simulink library "navigations"  (R2014a)
settings: Solver=ode45  StartTime=0.0  StopTime=10.0  RelTol=1e-3
undefined symbols (not defined in the file or in its folder): fdesignblkfcn, gcbh
libraries: simulink x8, visionstatistics x6
settings Model: Creator=jsustare  LastModifiedBy=jsustare

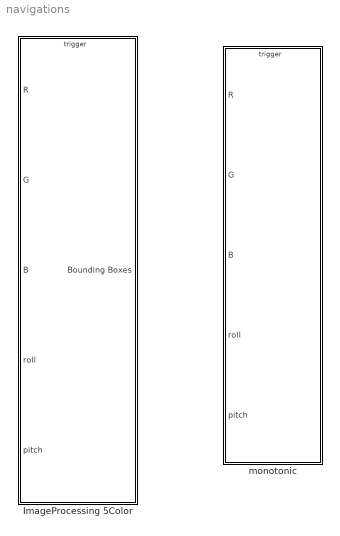
== system navigations ==
  ImageProcessing 5Color : Subsystem  TreatAsAtomicUnit=on  mask{blueThreshold=15, redThreshold=50, greenThreshold=50, yellowThreshold=160, purpleThreshold=160}
  monotonic : Subsystem  mask{whiteThreshold=0}
      mask prompts: whiteThreshold "whyite"

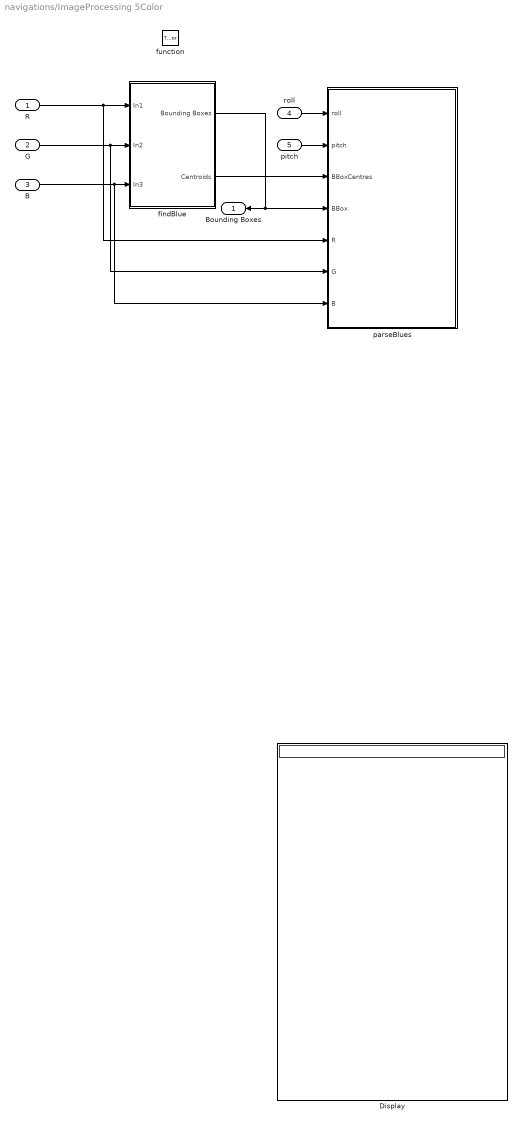
== system navigations/ImageProcessing 5Color ==
  R : Inport
  G : Inport  Port=2
  B : Inport  Port=3
  roll : Inport  Port=4
  pitch : Inport  Port=5
  function : TriggerPort  TriggerType=function-call
  Display : Display
  findBlue : Subsystem
  parseBlues : Subsystem  TreatAsAtomicUnit=on
  "Bounding Boxes " : Outport
  wires:
  pitch/1 -> parseBlues/2(pitch)
  roll/1 -> parseBlues/1(roll)
  findBlue/2(Centroids) -> parseBlues/3(BBoxCentres)
  findBlue/1(Bounding Boxes) -> "Bounding Boxes "/1, parseBlues/4(BBox)
  B/1 -> findBlue/3(In3), parseBlues/7(B)
  R/1 -> findBlue/1(In1), parseBlues/5(R)
  G/1 -> findBlue/2(In2), parseBlues/6(G)

== system navigations/monotonic ==
  note: use the writePos to store final positions per
      | landmark. keep inmind that this is suppose to
      |  beinside a loop and then the -1 scenarious would
      |  leand to -1000 cases
  R : Inport
  G : Inport  Port=2
  B : Inport  Port=3
  roll : Inport  Port=4
  pitch : Inport  Port=5
  function : TriggerPort  TriggerType=function-call
  MATLAB Function2 : MATLAB Function  TreatAsAtomicUnit=on
  detectLandMarks : Subsystem
  getPosition : Subsystem
  wires:
  R/1 -> detectLandMarks/1(R)
  B/1 -> detectLandMarks/3(B)
  G/1 -> detectLandMarks/2(G)

== system navigations/ImageProcessing 5Color/findBlue ==
  In1 : Inport
  In2 : Inport  Port=2
  In3 : Inport  Port=3
  Blob Analysis : visionstatistics/Blob Analysis  Tag=vipblks_row_conv  area=on  centroid=on  bBox=on  majorAxis=off  minorAxis=off  angle=off  eccentricity=off  equivDiameterSq=off  extent=off  perimeter=off  maxBlobs=16  warnIfNumBlobsExceeded=on  isCount=off  useMinArea=on  minArea=300  useMaxArea=off  maxArea=intmax('uint32')  excludeBorderBlob=on  outDT=double  isOutVarDim=off  isFill=on  fillValues=-1  conn=8  isLabel=off  outputMode=Binary point scaling  outputWordLength=32  outputFracLength=16  firstCoeffMode=Binary point scaling  firstCoeffWordLength=16  firstCoeffFracLength=14  secondCoeffMode=Binary point scaling  secondCoeffWordLength=32  secondCoeffFracLength=16  accumMode=Binary point scaling  accumWordLength=32  accumFracLength=0  prodOutputMode=Binary point scaling  prodOutputWordLength=32  prodOutputFracLength=16  roundingMode=Floor  overflowMode=off
  Compare To Constant : simulink/Logic and Bit Operations/Compare To Constant  relop=>  const=blueThreshold  OutDataTypeStr=boolean
  MATLAB Function : MATLAB Function  TreatAsAtomicUnit=on
  MATLAB Function1 : MATLAB Function  TreatAsAtomicUnit=on
  Bounding Boxes : Outport
  Centroids : Outport  Port=2
  wires:
  In3/1 -> MATLAB Function1/3(B)
  In2/1 -> MATLAB Function1/2(G)
  In1/1 -> MATLAB Function1/1(R)
  MATLAB Function1/1(blueIntensity) -> Compare To Constant/1
  Blob Analysis/2 -> MATLAB Function/2(centroid)
  MATLAB Function/1(centroid_largest) -> Centroids/1
  MATLAB Function/2(bbox_largest) -> Bounding Boxes/1
  Blob Analysis/1 -> MATLAB Function/1(area)
  Blob Analysis/3 -> MATLAB Function/3(bbox)
  Compare To Constant/1 -> Blob Analysis/1

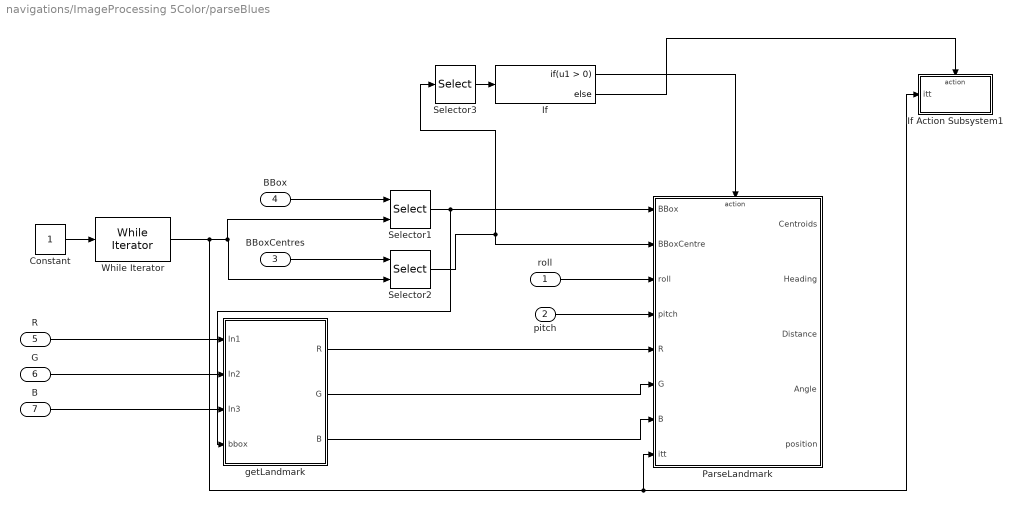
== system navigations/ImageProcessing 5Color/parseBlues ==
  roll : Inport
  pitch : Inport  Port=2
  BBoxCentres : Inport  Port=3
  BBox : Inport  Port=4
  R : Inport  Port=5
  G : Inport  Port=6
  B : Inport  Port=7
  Constant : Constant
  If : If
  If Action Subsystem1 : Subsystem  TreatAsAtomicUnit=on
  ParseLandmark : Subsystem  TreatAsAtomicUnit=on
  Selector1 : Selector  NumberOfDimensions=2  InputPortWidth=3  IndexOptions=Index vector (port),Select all  Indices=[1 3],1  OutputSizes=1,1
  Selector2 : Selector  NumberOfDimensions=2  InputPortWidth=3  IndexOptions=Index vector (port),Select all  Indices=[1 3],1  OutputSizes=1,1
  Selector3 : Selector  InputPortWidth=2
  While Iterator : WhileIterator  MaxIters=4  WhileBlockType=do-while  ShowIterationPort=on
  getLandmark : Subsystem
  wires:
  Selector3/1 -> If/1
  If/2 -> If Action Subsystem1/Action
  If/1 -> ParseLandmark/Action
  getLandmark/3(B) -> ParseLandmark/7(B)
  getLandmark/2(G) -> ParseLandmark/6(G)
  getLandmark/1(R) -> ParseLandmark/5(R)
  Constant/1 -> While Iterator/1
  B/1 -> getLandmark/3(In3)
  G/1 -> getLandmark/2(In2)
  R/1 -> getLandmark/1(In1)
  Selector2/1 -> ParseLandmark/2(BBoxCentre), Selector3/1
  Selector1/1 -> getLandmark/4(bbox), ParseLandmark/1(BBox)
  BBoxCentres/1 -> Selector2/1
  BBox/1 -> Selector1/1
  While Iterator/1 -> Selector2/2, Selector1/2, If Action Subsystem1/1(itt), ParseLandmark/8("itt ")
  pitch/1 -> ParseLandmark/4(pitch)
  roll/1 -> ParseLandmark/3(roll)

== system navigations/monotonic/detectLandMarks ==
  R : Inport
  G : Inport  Port=2
  B : Inport  Port=3
  Blob Analysis : visionstatistics/Blob Analysis  Tag=vipblks_row_conv  area=on  centroid=on  bBox=off  majorAxis=off  minorAxis=off  angle=off  eccentricity=off  equivDiameterSq=off  extent=off  perimeter=off  maxBlobs=16  warnIfNumBlobsExceeded=on  isCount=off  useMinArea=on  minArea=300  useMaxArea=off  maxArea=intmax('uint32')  excludeBorderBlob=on  outDT=double  isOutVarDim=off  isFill=on  fillValues=-1  conn=8  isLabel=off  outputMode=Binary point scaling  outputWordLength=32  outputFracLength=16  firstCoeffMode=Binary point scaling  firstCoeffWordLength=16  firstCoeffFracLength=14  secondCoeffMode=Binary point scaling  secondCoeffWordLength=32  secondCoeffFracLength=16  accumMode=Binary point scaling  accumWordLength=32  accumFracLength=0  prodOutputMode=Binary point scaling  prodOutputWordLength=32  prodOutputFracLength=16  roundingMode=Floor  overflowMode=off
  Compare To Constant : simulink/Logic and Bit Operations/Compare To Constant  relop=>  const=whiteThreshold  OutDataTypeStr=boolean
  MATLAB Function1 : MATLAB Function  TreatAsAtomicUnit=on
  MATLAB Function2 : MATLAB Function  TreatAsAtomicUnit=on
  centroids : Outport
  areas : Outport  Port=2
  wires:
  MATLAB Function1/2(areas_largest) -> areas/1
  MATLAB Function1/1(centroid_largest) -> centroids/1
  MATLAB Function2/1(whiteIntensity) -> Compare To Constant/1
  Blob Analysis/2 -> MATLAB Function1/2(centroid)
  Blob Analysis/1 -> MATLAB Function1/1(area)
  Compare To Constant/1 -> Blob Analysis/1
  B/1 -> MATLAB Function2/3(B)
  G/1 -> MATLAB Function2/2(G)
  R/1 -> MATLAB Function2/1(R)

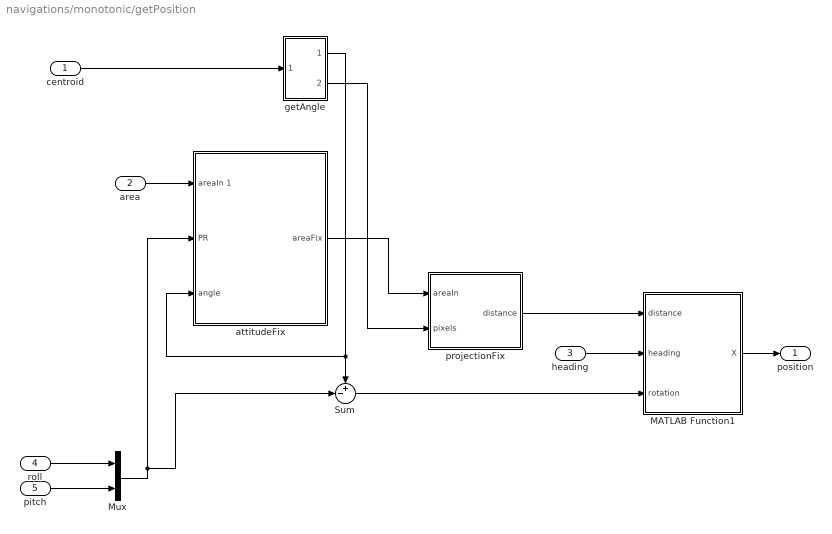
== system navigations/monotonic/getPosition ==
  centroid : Inport
  area : Inport  Port=2
  heading : Inport  Port=3
  "roll " : Inport  Port=4
  pitch : Inport  Port=5
  MATLAB Function1 : MATLAB Function  TreatAsAtomicUnit=on
  Mux : Mux  Inputs=2
  Sum : Sum  Inputs=+-|
  attitudeFix : Subsystem
  getAngle : Subsystem
  projectionFix : Subsystem
  position : Outport
  wires:
  getAngle/2(pixels) -> projectionFix/2(pixels)
  area/1 -> attitudeFix/1(areaIn 1)
  MATLAB Function1/1(X) -> position/1
  heading/1 -> MATLAB Function1/2(heading)
  projectionFix/1(distance) -> MATLAB Function1/1(distance)
  attitudeFix/1(areaFix) -> projectionFix/1(areaIn)
  Sum/1 -> MATLAB Function1/3(rotation)
  getAngle/1(angleRad) -> Sum/1, attitudeFix/3("angle ")
  Mux/1 -> Sum/2, attitudeFix/2(PR)
  pitch/1 -> Mux/2
  "roll "/1 -> Mux/1
  centroid/1 -> getAngle/1(centroid)

== system navigations/ImageProcessing 5Color/parseBlues/If Action Subsystem1 ==
  itt : Inport
  Action Port : ActionPort
  MATLAB Function1 : MATLAB Function  TreatAsAtomicUnit=on
  wires:
  itt/1 -> MATLAB Function1/1(itt)

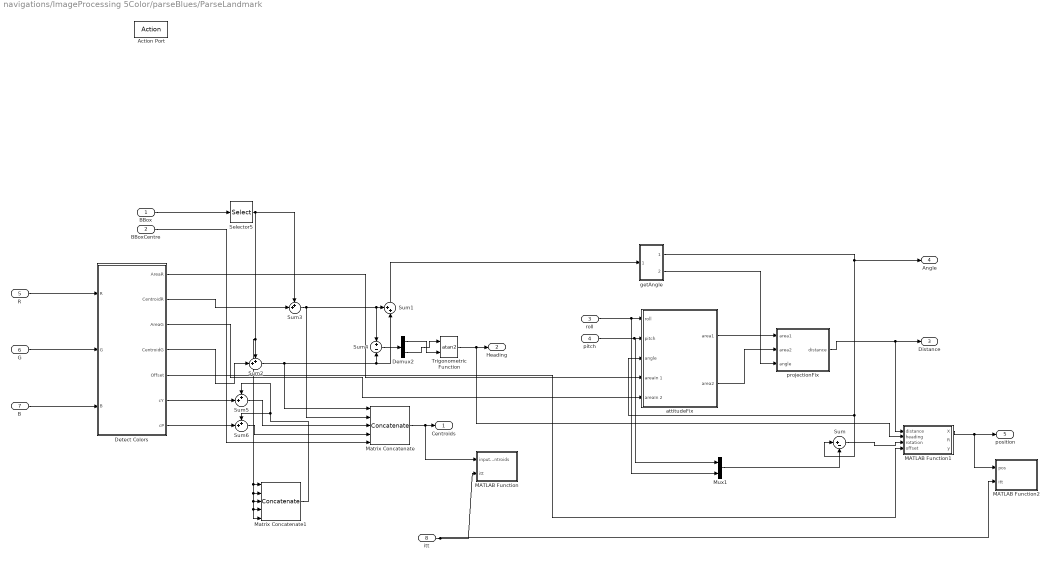
== system navigations/ImageProcessing 5Color/parseBlues/ParseLandmark ==
  BBox : Inport
  BBoxCentre : Inport  Port=2
  roll : Inport  Port=3
  pitch : Inport  Port=4
  R : Inport  Port=5
  G : Inport  Port=6
  B : Inport  Port=7
  "itt " : Inport  Port=8
  Action Port : ActionPort  PropagateVarSize=During execution
  Demux2 : Demux  Outputs=2
  Detect Colors : Subsystem
  MATLAB Function : MATLAB Function  TreatAsAtomicUnit=on
  MATLAB Function1 : MATLAB Function  TreatAsAtomicUnit=on
  MATLAB Function2 : MATLAB Function  TreatAsAtomicUnit=on
  Matrix Concatenate : Concatenate  NumInputs=5  Mode=Multidimensional array
  Matrix Concatenate1 : Concatenate  NumInputs=5  Mode=Multidimensional array
  Mux1 : Mux  Inputs=2
  Selector5 : Selector  InputPortWidth=4  Indices=[1 2]
  Sum : Sum  Inputs=|+-
  Sum{1..3,5..6} (5 alike) : Sum  Inputs=++|
  Sum4 : Sum  Inputs=+-
  Trigonometric Function : Trigonometry  Operator=atan2
  attitudeFix : Subsystem
  getAngle : Subsystem
  projectionFix : Subsystem
  Centroids : Outport
  Heading : Outport  Port=2
  "Distance " : Outport  Port=3
  Angle : Outport  Port=4
  position : Outport  Port=5
  wires:
  getAngle/2(Out2) -> projectionFix/3(angle)
  Sum1/1 -> getAngle/1(In1)
  getAngle/1(Out1) -> Angle/1, Sum/1, attitudeFix/3("angle ")
  "itt "/1 -> MATLAB Function/2(itt), MATLAB Function2/2(itt)
  Matrix Concatenate/1 -> Centroids/1, MATLAB Function/1(inputCentroids)
  pitch/1 -> Mux1/1, attitudeFix/2(pitch)
  attitudeFix/1(area1) -> projectionFix/1(area1)
  attitudeFix/2(area2) -> projectionFix/2(area2)
  Sum4/1 -> Demux2/1
  Demux2/2 -> Trigonometric Function/1
  Demux2/1 -> Trigonometric Function/2
  Detect Colors/2(CentroidR) -> Sum3/2
  Sum3/1 -> Matrix Concatenate/2, Sum1/1, Sum4/1
  Detect Colors/1(AreaR) -> attitudeFix/4(areaIn 1)
  projectionFix/1(distance) -> MATLAB Function1/1(distance), "Distance "/1
  BBox/1 -> Selector5/1
  Detect Colors/4(CentroidG) -> Sum2/2
  Sum2/1 -> Matrix Concatenate/1, Sum1/2, Sum4/2
  Detect Colors/3(AreaG) -> attitudeFix/5(areaIn 2)
  Sum/1 -> MATLAB Function1/3(rotation)
  Mux1/1 -> Sum/2
  roll/1 -> Mux1/2, attitudeFix/1(roll)
  Trigonometric Function/1 -> MATLAB Function1/2(heading), Heading/1
  MATLAB Function1/1(X) -> position/1, MATLAB Function2/1(pos)
  Detect Colors/6(cY) -> Sum5/2
  Detect Colors/7(cP) -> Sum6/2
  Sum6/1 -> Matrix Concatenate/4
  Sum5/1 -> Matrix Concatenate/3
  BBoxCentre/1 -> Matrix Concatenate/5
  Selector5/1 -> Sum3/1, Matrix Concatenate1/1, Matrix Concatenate1/2, Matrix Concatenate1/3, Matrix Concatenate1/4, Matrix Concatenate1/5, Sum2/1
  Matrix Concatenate1/1 -> Sum6/1, Sum5/1
  R/1 -> Detect Colors/1(R)
  G/1 -> Detect Colors/2(G)
  B/1 -> Detect Colors/3(B)
  Detect Colors/5(Offset) -> MATLAB Function1/4(offset)

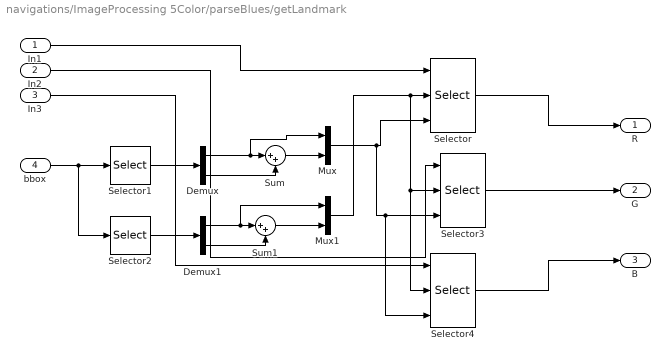
== system navigations/ImageProcessing 5Color/parseBlues/getLandmark ==
  In1 : Inport
  In2 : Inport  Port=2
  In3 : Inport  Port=3
  bbox : Inport  Port=4
  Demux : Demux  Outputs=2
  Demux1 : Demux  Outputs=2
  Mux : Mux  Inputs=2
  Mux1 : Mux  Inputs=2
  Selector : Selector  NumberOfDimensions=2  InputPortWidth=3  IndexOptions=Starting and ending indices (port),Starting and ending indices (port)  Indices=[1 3],1  OutputSizes=1,1
  Selector1 : Selector  InputPortWidth=4  Indices=[1 3]
  Selector2 : Selector  InputPortWidth=4  Indices=[2 4]
  Selector3 : Selector  NumberOfDimensions=2  InputPortWidth=3  IndexOptions=Starting and ending indices (port),Starting and ending indices (port)  Indices=[1 3],1  OutputSizes=1,1
  Selector4 : Selector  NumberOfDimensions=2  InputPortWidth=3  IndexOptions=Starting and ending indices (port),Starting and ending indices (port)  Indices=[1 3],1  OutputSizes=1,1
  Sum : Sum  Inputs=|++
  Sum1 : Sum  Inputs=|++
  R : Outport
  G : Outport  Port=2
  B : Outport  Port=3
  wires:
  Mux1/1 -> Selector/2, Selector3/2, Selector4/2
  Mux/1 -> Selector/3, Selector3/3, Selector4/3
  Selector4/1 -> B/1
  Selector3/1 -> G/1
  Selector/1 -> R/1
  Sum1/1 -> Mux1/2
  Sum/1 -> Mux/2
  Demux1/2 -> Sum1/2
  Demux1/1 -> Sum1/1, Mux1/1
  Demux/2 -> Sum/2
  Demux/1 -> Sum/1, Mux/1
  Selector2/1 -> Demux1/1
  Selector1/1 -> Demux/1
  bbox/1 -> Selector1/1, Selector2/1
  In3/1 -> Selector4/1
  In2/1 -> Selector3/1
  In1/1 -> Selector/1

== system navigations/monotonic/getPosition/attitudeFix ==
  areaIn 1 : Inport
  PR : Inport  Port=2
  "angle " : Inport  Port=3
  Constant : Constant
  MATLAB Function : MATLAB Function  TreatAsAtomicUnit=on
  Math Function : Math  Operator=pow  SaturateOnIntegerOverflow=on
  Product1 : Product
  areaFix : Outport
  wires:
  Math Function/1 -> Product1/1
  Constant/1 -> Math Function/2
  MATLAB Function/1(c) -> Math Function/1
  areaIn 1/1 -> Product1/2
  Product1/1 -> areaFix/1
  "angle "/1 -> MATLAB Function/2(angle)
  PR/1 -> MATLAB Function/1(PR)

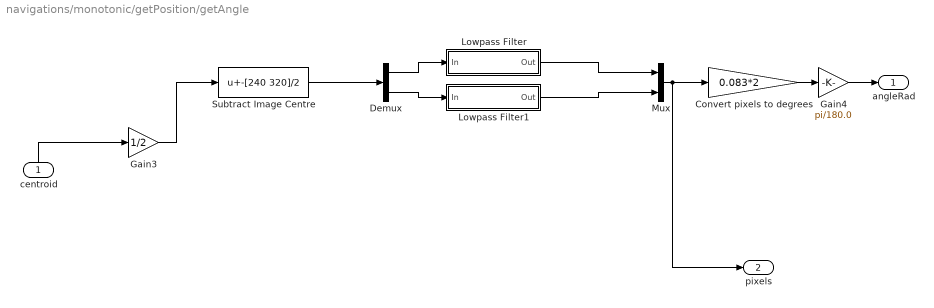
== system navigations/monotonic/getPosition/getAngle ==
  centroid : Inport
  Convert pixels to degrees : Gain  Gain=0.083*2
  Demux : Demux  Outputs=2
  Gain3 : Gain  Gain=1/2
  Gain4 : Gain  Gain=pi/180.0
  Lowpass Filter : Subsystem  DialogController=fdesignblkfcn  InitFcn=fdesignblkfcn(gcbh, {'InitFcn'});  mask(Lowpass Filter){}
      mask help: Design a lowpass filter
      settings: CopyFcn=fdesignblkfcn(gcbh, {'CopyFcn'});
      mask Help: helpview(mapfilelocation('dsp'), 'dsplowpassfilter');
      mask Display: disp('Lowpass')
  Lowpass Filter1 : Subsystem  DialogController=fdesignblkfcn  InitFcn=fdesignblkfcn(gcbh, {'InitFcn'});  mask(Lowpass Filter){}
      mask help: Design a lowpass filter
      settings: CopyFcn=fdesignblkfcn(gcbh, {'CopyFcn'});
      mask Help: helpview(mapfilelocation('dsp'), 'dsplowpassfilter');
      mask Display: disp('Lowpass')
  Mux : Mux  Inputs=2
  Subtract Image Centre : Bias  Bias=-[240 320]/2
  angleRad : Outport
  pixels : Outport  Port=2
  wires:
  Gain4/1 -> angleRad/1
  Convert pixels to degrees/1 -> Gain4/1
  Subtract Image Centre/1 -> Demux/1
  Gain3/1 -> Subtract Image Centre/1
  centroid/1 -> Gain3/1
  Lowpass Filter1/1(Out) -> Mux/2
  Lowpass Filter/1(Out) -> Mux/1
  Demux/1 -> Lowpass Filter/1(In)
  Demux/2 -> Lowpass Filter1/1(In)
  Mux/1 -> pixels/1, Convert pixels to degrees/1

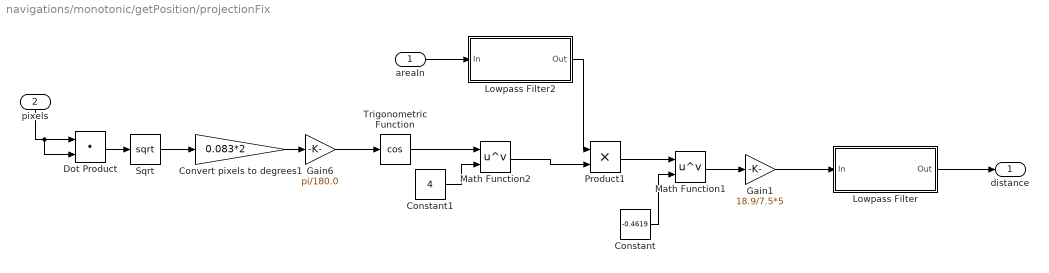
== system navigations/monotonic/getPosition/projectionFix ==
  areaIn : Inport
  pixels : Inport  Port=2
  Constant : Constant  Value=-0.4619
  Constant1 : Constant  Value=4
  Convert pixels to degrees1 : Gain  Gain=0.083*2
  Dot Product : DotProduct  InputSameDT=on  OutDataTypeStr=Inherit: Inherit via internal rule
  Gain1 : Gain  Gain=18.9/7.5*5
  Gain6 : Gain  Gain=pi/180.0
  Lowpass Filter : Subsystem  DialogController=fdesignblkfcn  InitFcn=fdesignblkfcn(gcbh, {'InitFcn'});  mask(Lowpass Filter){}
      mask help: Design a lowpass filter
      settings: CopyFcn=fdesignblkfcn(gcbh, {'CopyFcn'});
      mask Help: helpview(mapfilelocation('dsp'), 'dsplowpassfilter');
      mask Display: disp('Lowpass')
  Lowpass Filter2 : Subsystem  DialogController=fdesignblkfcn  InitFcn=fdesignblkfcn(gcbh, {'InitFcn'});  mask(Lowpass Filter){}
      mask help: Design a lowpass filter
      settings: CopyFcn=fdesignblkfcn(gcbh, {'CopyFcn'});
      mask Help: helpview(mapfilelocation('dsp'), 'dsplowpassfilter');
      mask Display: disp('Lowpass')
  Math Function1 : Math  Operator=pow  SaturateOnIntegerOverflow=on
  Math Function2 : Math  Operator=pow  SaturateOnIntegerOverflow=on
  Product1 : Product
  Sqrt : Sqrt  SaturateOnIntegerOverflow=on
  Trigonometric Function : Trigonometry  Operator=cos
  distance : Outport
  wires:
  Constant1/1 -> Math Function2/2
  Lowpass Filter2/1(Out) -> Product1/1
  Trigonometric Function/1 -> Math Function2/1
  Math Function2/1 -> Product1/2
  Product1/1 -> Math Function1/1
  Gain1/1 -> Lowpass Filter/1(In)
  Sqrt/1 -> Convert pixels to degrees1/1
  Dot Product/1 -> Sqrt/1
  Gain6/1 -> Trigonometric Function/1
  Convert pixels to degrees1/1 -> Gain6/1
  Lowpass Filter/1(Out) -> distance/1
  areaIn/1 -> Lowpass Filter2/1(In)
  Constant/1 -> Math Function1/2
  Math Function1/1 -> Gain1/1
  pixels/1 -> Dot Product/1, Dot Product/2

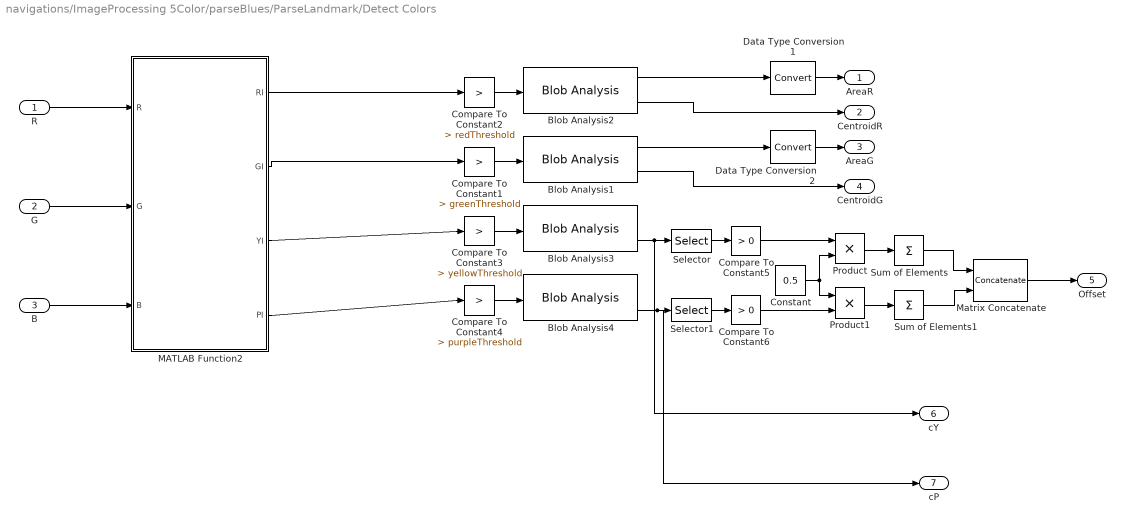
== system navigations/ImageProcessing 5Color/parseBlues/ParseLandmark/Detect Colors ==
  R : Inport
  G : Inport  Port=2
  B : Inport  Port=3
  Blob Analysis1 : visionstatistics/Blob Analysis  Tag=vipblks_row_conv  area=on  centroid=on  bBox=off  majorAxis=off  minorAxis=off  angle=off  eccentricity=off  equivDiameterSq=off  extent=off  perimeter=off  maxBlobs=1  warnIfNumBlobsExceeded=on  isCount=off  useMinArea=off  minArea=0  useMaxArea=off  maxArea=intmax('uint32')  excludeBorderBlob=off  outDT=double  isOutVarDim=off  isFill=on  fillValues=-1  conn=8  isLabel=off  outputMode=Binary point scaling  outputWordLength=32  outputFracLength=16  firstCoeffMode=Binary point scaling  firstCoeffWordLength=16  firstCoeffFracLength=14  secondCoeffMode=Binary point scaling  secondCoeffWordLength=32  secondCoeffFracLength=16  accumMode=Binary point scaling  accumWordLength=32  accumFracLength=0  prodOutputMode=Binary point scaling  prodOutputWordLength=32  prodOutputFracLength=16  roundingMode=Floor  overflowMode=off
  Blob Analysis2 : visionstatistics/Blob Analysis  Tag=vipblks_row_conv  area=on  centroid=on  bBox=off  majorAxis=off  minorAxis=off  angle=off  eccentricity=off  equivDiameterSq=off  extent=off  perimeter=off  maxBlobs=1  warnIfNumBlobsExceeded=on  isCount=off  useMinArea=off  minArea=0  useMaxArea=off  maxArea=intmax('uint32')  excludeBorderBlob=off  outDT=double  isOutVarDim=off  isFill=on  fillValues=-1  conn=8  isLabel=off  outputMode=Binary point scaling  outputWordLength=32  outputFracLength=16  firstCoeffMode=Binary point scaling  firstCoeffWordLength=16  firstCoeffFracLength=14  secondCoeffMode=Binary point scaling  secondCoeffWordLength=32  secondCoeffFracLength=16  accumMode=Binary point scaling  accumWordLength=32  accumFracLength=0  prodOutputMode=Binary point scaling  prodOutputWordLength=32  prodOutputFracLength=16  roundingMode=Floor  overflowMode=off
  Blob Analysis3 : visionstatistics/Blob Analysis  Tag=vipblks_row_conv  area=on  centroid=on  bBox=off  majorAxis=off  minorAxis=off  angle=off  eccentricity=off  equivDiameterSq=off  extent=off  perimeter=off  maxBlobs=5  warnIfNumBlobsExceeded=on  isCount=off  useMinArea=on  minArea=10  useMaxArea=off  maxArea=intmax('uint32')  excludeBorderBlob=off  outDT=double  isOutVarDim=off  isFill=on  fillValues=-1  conn=8  isLabel=off  outputMode=Binary point scaling  outputWordLength=32  outputFracLength=16  firstCoeffMode=Binary point scaling  firstCoeffWordLength=16  firstCoeffFracLength=14  secondCoeffMode=Binary point scaling  secondCoeffWordLength=32  secondCoeffFracLength=16  accumMode=Binary point scaling  accumWordLength=32  accumFracLength=0  prodOutputMode=Binary point scaling  prodOutputWordLength=32  prodOutputFracLength=16  roundingMode=Floor  overflowMode=off
  Blob Analysis4 : visionstatistics/Blob Analysis  Tag=vipblks_row_conv  area=on  centroid=on  bBox=off  majorAxis=off  minorAxis=off  angle=off  eccentricity=off  equivDiameterSq=off  extent=off  perimeter=off  maxBlobs=5  warnIfNumBlobsExceeded=on  isCount=off  useMinArea=on  minArea=10  useMaxArea=off  maxArea=intmax('uint32')  excludeBorderBlob=off  outDT=double  isOutVarDim=off  isFill=on  fillValues=-1  conn=8  isLabel=off  outputMode=Binary point scaling  outputWordLength=32  outputFracLength=16  firstCoeffMode=Binary point scaling  firstCoeffWordLength=16  firstCoeffFracLength=14  secondCoeffMode=Binary point scaling  secondCoeffWordLength=32  secondCoeffFracLength=16  accumMode=Binary point scaling  accumWordLength=32  accumFracLength=0  prodOutputMode=Binary point scaling  prodOutputWordLength=32  prodOutputFracLength=16  roundingMode=Floor  overflowMode=off
  Compare To Constant1 : simulink/Logic and Bit Operations/Compare To Constant  relop=>  const=greenThreshold  OutDataTypeStr=boolean
  Compare To Constant2 : simulink/Logic and Bit Operations/Compare To Constant  relop=>  const=redThreshold  OutDataTypeStr=boolean
  Compare To Constant3 : simulink/Logic and Bit Operations/Compare To Constant  relop=>  const=yellowThreshold  OutDataTypeStr=boolean
  Compare To Constant4 : simulink/Logic and Bit Operations/Compare To Constant  relop=>  const=purpleThreshold  OutDataTypeStr=boolean
  Compare To Constant5 : simulink/Logic and Bit Operations/Compare To Constant  relop=>  const=0  OutDataTypeStr=boolean
  Compare To Constant6 : simulink/Logic and Bit Operations/Compare To Constant  relop=>  const=0  OutDataTypeStr=boolean
  Constant : Constant  Value=0.5
  Data Type Conversion1 : DataTypeConversion
  Data Type Conversion2 : DataTypeConversion
  MATLAB Function2 : MATLAB Function  TreatAsAtomicUnit=on
  Matrix Concatenate : Concatenate  Mode=Multidimensional array  ConcatenateDimension=2
  Product : Product
  Product1 : Product
  Selector : Selector  NumberOfDimensions=2  InputPortWidth=3  IndexOptions=Select all,Index vector (dialog)  Indices=1,1  OutputSizes=1,1
  Selector1 : Selector  NumberOfDimensions=2  InputPortWidth=3  IndexOptions=Select all,Index vector (dialog)  Indices=1,1  OutputSizes=1,1
  Sum of Elements : Sum  Inputs=+
  Sum of Elements1 : Sum  Inputs=+
  AreaR : Outport
  CentroidR : Outport  Port=2
  AreaG : Outport  Port=3
  CentroidG : Outport  Port=4
  Offset : Outport  Port=5
  cY : Outport  Port=6
  cP : Outport  Port=7
  wires:
  MATLAB Function2/1(RI) -> Compare To Constant2/1
  Compare To Constant2/1 -> Blob Analysis2/1
  Blob Analysis2/2 -> CentroidR/1
  Blob Analysis2/1 -> Data Type Conversion1/1
  Data Type Conversion1/1 -> AreaR/1
  Compare To Constant1/1 -> Blob Analysis1/1
  Blob Analysis1/2 -> CentroidG/1
  Blob Analysis1/1 -> Data Type Conversion2/1
  Data Type Conversion2/1 -> AreaG/1
  MATLAB Function2/2(GI) -> Compare To Constant1/1
  Compare To Constant3/1 -> Blob Analysis3/1
  MATLAB Function2/3(YI) -> Compare To Constant3/1
  Compare To Constant4/1 -> Blob Analysis4/1
  MATLAB Function2/4(PI) -> Compare To Constant4/1
  Blob Analysis3/2 -> cY/1, Selector/1
  Blob Analysis4/2 -> cP/1, Selector1/1
  Selector/1 -> Compare To Constant5/1
  Selector1/1 -> Compare To Constant6/1
  Compare To Constant5/1 -> Product/1
  Compare To Constant6/1 -> Product1/2
  Constant/1 -> Product1/1, Product/2
  Product/1 -> Sum of Elements/1
  Product1/1 -> Sum of Elements1/1
  Sum of Elements/1 -> Matrix Concatenate/1
  Sum of Elements1/1 -> Matrix Concatenate/2
  Matrix Concatenate/1 -> Offset/1
  R/1 -> MATLAB Function2/1(R)
  G/1 -> MATLAB Function2/2(G)
  B/1 -> MATLAB Function2/3(B)

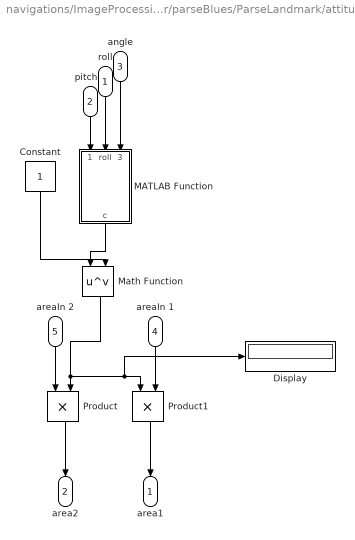
== system navigations/ImageProcessing 5Color/parseBlues/ParseLandmark/attitudeFix ==
  roll : Inport
  pitch : Inport  Port=2
  "angle " : Inport  Port=3
  areaIn 1 : Inport  Port=4
  areaIn 2 : Inport  Port=5
  Constant : Constant
  Display : Display
  MATLAB Function : MATLAB Function  TreatAsAtomicUnit=on
  Math Function : Math  Operator=pow  SaturateOnIntegerOverflow=on
  Product : Product
  Product1 : Product
  area1 : Outport
  area2 : Outport  Port=2
  wires:
  pitch/1 -> MATLAB Function/1(pitch)
  roll/1 -> MATLAB Function/2(roll)
  "angle "/1 -> MATLAB Function/3(angle)
  Product1/1 -> area1/1
  Product/1 -> area2/1
  areaIn 2/1 -> Product/1
  areaIn 1/1 -> Product1/2
  MATLAB Function/1(c) -> Math Function/1
  Constant/1 -> Math Function/2
  Math Function/1 -> Display/1, Product1/1, Product/2

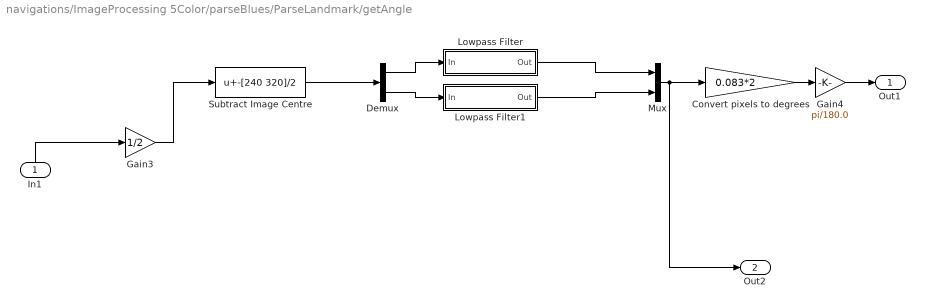
== system navigations/ImageProcessing 5Color/parseBlues/ParseLandmark/getAngle ==
  In1 : Inport
  Convert pixels to degrees : Gain  Gain=0.083*2
  Demux : Demux  Outputs=2
  Gain3 : Gain  Gain=1/2
  Gain4 : Gain  Gain=pi/180.0
  Lowpass Filter : Subsystem  DialogController=fdesignblkfcn  InitFcn=fdesignblkfcn(gcbh, {'InitFcn'});  mask(Lowpass Filter){}
      mask help: Design a lowpass filter
      settings: CopyFcn=fdesignblkfcn(gcbh, {'CopyFcn'});
      mask Help: helpview(mapfilelocation('dsp'), 'dsplowpassfilter');
      mask Display: disp('Lowpass')
  Lowpass Filter1 : Subsystem  DialogController=fdesignblkfcn  InitFcn=fdesignblkfcn(gcbh, {'InitFcn'});  mask(Lowpass Filter){}
      mask help: Design a lowpass filter
      settings: CopyFcn=fdesignblkfcn(gcbh, {'CopyFcn'});
      mask Help: helpview(mapfilelocation('dsp'), 'dsplowpassfilter');
      mask Display: disp('Lowpass')
  Mux : Mux  Inputs=2
  Subtract Image Centre : Bias  Bias=-[240 320]/2
  Out1 : Outport
  Out2 : Outport  Port=2
  wires:
  Mux/1 -> Convert pixels to degrees/1, Out2/1
  Demux/2 -> Lowpass Filter1/1(In)
  Demux/1 -> Lowpass Filter/1(In)
  Lowpass Filter/1(Out) -> Mux/1
  Lowpass Filter1/1(Out) -> Mux/2
  In1/1 -> Gain3/1
  Gain3/1 -> Subtract Image Centre/1
  Subtract Image Centre/1 -> Demux/1
  Convert pixels to degrees/1 -> Gain4/1
  Gain4/1 -> Out1/1

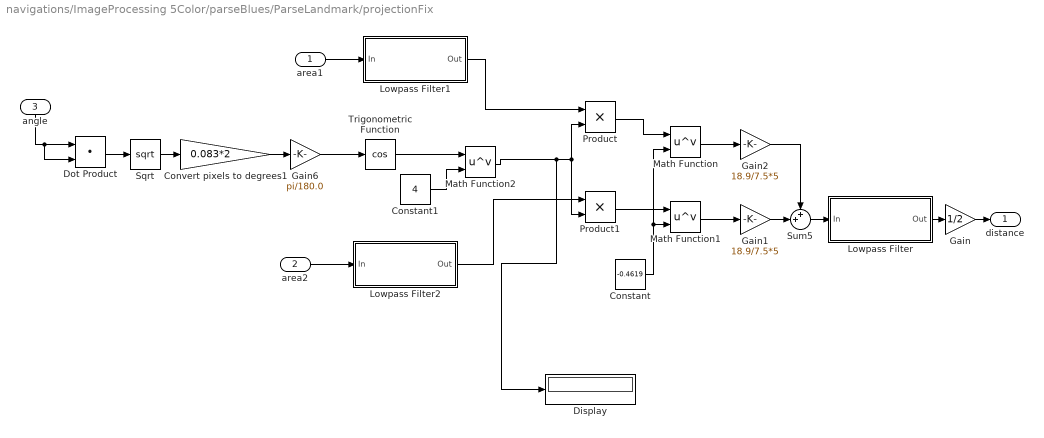
== system navigations/ImageProcessing 5Color/parseBlues/ParseLandmark/projectionFix ==
  area1 : Inport
  area2 : Inport  Port=2
  angle : Inport  Port=3
  Constant : Constant  Value=-0.4619
  Constant1 : Constant  Value=4
  Convert pixels to degrees1 : Gain  Gain=0.083*2
  Display : Display
  Dot Product : DotProduct  InputSameDT=on  OutDataTypeStr=Inherit: Inherit via internal rule
  Gain : Gain  Gain=1/2
  Gain1 : Gain  Gain=18.9/7.5*5
  Gain2 : Gain  Gain=18.9/7.5*5
  Gain6 : Gain  Gain=pi/180.0
  Lowpass Filter : Subsystem  DialogController=fdesignblkfcn  InitFcn=fdesignblkfcn(gcbh, {'InitFcn'});  mask(Lowpass Filter){}
      mask help: Design a lowpass filter
      settings: CopyFcn=fdesignblkfcn(gcbh, {'CopyFcn'});
      mask Help: helpview(mapfilelocation('dsp'), 'dsplowpassfilter');
      mask Display: disp('Lowpass')
  Lowpass Filter1 : Subsystem  DialogController=fdesignblkfcn  InitFcn=fdesignblkfcn(gcbh, {'InitFcn'});  mask(Lowpass Filter){}
      mask help: Design a lowpass filter
      settings: CopyFcn=fdesignblkfcn(gcbh, {'CopyFcn'});
      mask Help: helpview(mapfilelocation('dsp'), 'dsplowpassfilter');
      mask Display: disp('Lowpass')
  Lowpass Filter2 : Subsystem  DialogController=fdesignblkfcn  InitFcn=fdesignblkfcn(gcbh, {'InitFcn'});  mask(Lowpass Filter){}
      mask help: Design a lowpass filter
      settings: CopyFcn=fdesignblkfcn(gcbh, {'CopyFcn'});
      mask Help: helpview(mapfilelocation('dsp'), 'dsplowpassfilter');
      mask Display: disp('Lowpass')
  Math Function : Math  Operator=pow  SaturateOnIntegerOverflow=on
  Math Function1 : Math  Operator=pow  SaturateOnIntegerOverflow=on
  Math Function2 : Math  Operator=pow  SaturateOnIntegerOverflow=on
  Product : Product
  Product1 : Product
  Sqrt : Sqrt  SaturateOnIntegerOverflow=on
  Sum5 : Sum  Inputs=++|
  Trigonometric Function : Trigonometry  Operator=cos
  distance : Outport
  wires:
  angle/1 -> Dot Product/2, Dot Product/1
  Math Function1/1 -> Gain1/1
  Math Function/1 -> Gain2/1
  Constant/1 -> Math Function/2, Math Function1/2
  area1/1 -> Lowpass Filter1/1(In)
  area2/1 -> Lowpass Filter2/1(In)
  Gain/1 -> distance/1
  Gain2/1 -> Sum5/1
  Gain1/1 -> Sum5/2
  Lowpass Filter/1(Out) -> Gain/1
  Convert pixels to degrees1/1 -> Gain6/1
  Gain6/1 -> Trigonometric Function/1
  Dot Product/1 -> Sqrt/1
  Sqrt/1 -> Convert pixels to degrees1/1
  Sum5/1 -> Lowpass Filter/1(In)
  Product/1 -> Math Function/1
  Product1/1 -> Math Function1/1
  Math Function2/1 -> Display/1, Product/2, Product1/2
  Trigonometric Function/1 -> Math Function2/1
  Lowpass Filter1/1(Out) -> Product/1
  Lowpass Filter2/1(Out) -> Product1/1
  Constant1/1 -> Math Function2/2

== system navigations/monotonic/getPosition/getAngle/Lowpass Filter ==
  In : Inport
  Generated Filter Block : DiscreteFir  Tag=BlockMethodSubSystem  Coefficients=[0.0032276888738420255 -0.012093185057654832 -0.056871256727662273 -0.033025317279675399 0.16717851315296134 0.40566714821275895 0.40566714821275895 0.16717851315296134 -0.033025317279675399 -0.056871256727662273 -0.012093185057654832 0.0032276888738420255]  InputProcessing=Columns as channels (frame based)
  Out : Outport
  wires:
  Generated Filter Block/1 -> Out/1
  In/1 -> Generated Filter Block/1

== system navigations/monotonic/getPosition/getAngle/Lowpass Filter1 ==
  In : Inport
  Generated Filter Block : DiscreteFir  Tag=BlockMethodSubSystem  Coefficients=[0.0032276888738420255 -0.012093185057654832 -0.056871256727662273 -0.033025317279675399 0.16717851315296134 0.40566714821275895 0.40566714821275895 0.16717851315296134 -0.033025317279675399 -0.056871256727662273 -0.012093185057654832 0.0032276888738420255]  InputProcessing=Columns as channels (frame based)
  Out : Outport
  wires:
  In/1 -> Generated Filter Block/1
  Generated Filter Block/1 -> Out/1

== system navigations/monotonic/getPosition/projectionFix/Lowpass Filter ==
  In : Inport
  Generated Filter Block : DiscreteFir  Tag=BlockMethodSubSystem  Coefficients=[0.011901508381575016 0.02908797826733928 0.0025913585662860131 -0.068996275507793012 -0.050025679925086837 0.16540100530640869 0.41332778671981452 0.41332778671981452 0.16540100530640869 -0.050025679925086837 -0.068996275507793012 0.0025913585662860131 0.02908797826733928 0.011901508381575016]  InputProcessing=Columns as channels (frame based)
  Out : Outport
  wires:
  Generated Filter Block/1 -> Out/1
  In/1 -> Generated Filter Block/1

== system navigations/monotonic/getPosition/projectionFix/Lowpass Filter2 ==
  In : Inport
  Generated Filter Block : DiscreteFir  Tag=BlockMethodSubSystem  Coefficients=[0.011901508381575016 0.02908797826733928 0.0025913585662860131 -0.068996275507793012 -0.050025679925086837 0.16540100530640869 0.41332778671981452 0.41332778671981452 0.16540100530640869 -0.050025679925086837 -0.068996275507793012 0.0025913585662860131 0.02908797826733928 0.011901508381575016]  InputProcessing=Columns as channels (frame based)
  Out : Outport
  wires:
  Generated Filter Block/1 -> Out/1
  In/1 -> Generated Filter Block/1

== system navigations/ImageProcessing 5Color/parseBlues/ParseLandmark/getAngle/Lowpass Filter ==
  In : Inport
  Generated Filter Block : DiscreteFir  Tag=BlockMethodSubSystem  Coefficients=[0.0032276888738420255 -0.012093185057654832 -0.056871256727662273 -0.033025317279675399 0.16717851315296134 0.40566714821275895 0.40566714821275895 0.16717851315296134 -0.033025317279675399 -0.056871256727662273 -0.012093185057654832 0.0032276888738420255]  InputProcessing=Columns as channels (frame based)
  Out : Outport
  wires:
  In/1 -> Generated Filter Block/1
  Generated Filter Block/1 -> Out/1

== system navigations/ImageProcessing 5Color/parseBlues/ParseLandmark/getAngle/Lowpass Filter1 ==
  In : Inport
  Generated Filter Block : DiscreteFir  Tag=BlockMethodSubSystem  Coefficients=[0.0032276888738420255 -0.012093185057654832 -0.056871256727662273 -0.033025317279675399 0.16717851315296134 0.40566714821275895 0.40566714821275895 0.16717851315296134 -0.033025317279675399 -0.056871256727662273 -0.012093185057654832 0.0032276888738420255]  InputProcessing=Columns as channels (frame based)
  Out : Outport
  wires:
  Generated Filter Block/1 -> Out/1
  In/1 -> Generated Filter Block/1

== system navigations/ImageProcessing 5Color/parseBlues/ParseLandmark/projectionFix/Lowpass Filter ==
  In : Inport
  Generated Filter Block : DiscreteFir  Tag=BlockMethodSubSystem  Coefficients=[0.011901508381575016 0.02908797826733928 0.0025913585662860131 -0.068996275507793012 -0.050025679925086837 0.16540100530640869 0.41332778671981452 0.41332778671981452 0.16540100530640869 -0.050025679925086837 -0.068996275507793012 0.0025913585662860131 0.02908797826733928 0.011901508381575016]  InputProcessing=Columns as channels (frame based)
  Out : Outport
  wires:
  In/1 -> Generated Filter Block/1
  Generated Filter Block/1 -> Out/1

== system navigations/ImageProcessing 5Color/parseBlues/ParseLandmark/projectionFix/Lowpass Filter1 ==
  In : Inport
  Generated Filter Block : DiscreteFir  Tag=BlockMethodSubSystem  Coefficients=[0.011901508381575016 0.02908797826733928 0.0025913585662860131 -0.068996275507793012 -0.050025679925086837 0.16540100530640869 0.41332778671981452 0.41332778671981452 0.16540100530640869 -0.050025679925086837 -0.068996275507793012 0.0025913585662860131 0.02908797826733928 0.011901508381575016]  InputProcessing=Columns as channels (frame based)
  Out : Outport
  wires:
  Generated Filter Block/1 -> Out/1
  In/1 -> Generated Filter Block/1

== system navigations/ImageProcessing 5Color/parseBlues/ParseLandmark/projectionFix/Lowpass Filter2 ==
  In : Inport
  Generated Filter Block : DiscreteFir  Tag=BlockMethodSubSystem  Coefficients=[0.011901508381575016 0.02908797826733928 0.0025913585662860131 -0.068996275507793012 -0.050025679925086837 0.16540100530640869 0.41332778671981452 0.41332778671981452 0.16540100530640869 -0.050025679925086837 -0.068996275507793012 0.0025913585662860131 0.02908797826733928 0.011901508381575016]  InputProcessing=Columns as channels (frame based)
  Out : Outport
  wires:
  In/1 -> Generated Filter Block/1
  Generated Filter Block/1 -> Out/1

== matlab function navigations/monotonic/MATLAB Function2 ==
  data: pos input; itt input; positionData data_store_memory
function writePos(pos, itt)
global positionData;
positionData(itt,:)=pos;

== matlab function navigations/monotonic/detectLandMarks/MATLAB Function1 ==
  data: area input; centroid_largest output; centroid input; areas_largest output
function [centroid_largest,areas_largest] = selectLargest(area, centroid)
[y, i] = sort(area);
l=length(area);
centroid_largest = [centroid(i(l),:); centroid(i(l-1),:) ;centroid(i(l-2),:);centroid(i(l-3),:) ];
centroid_largest = [area(i(l),:); area(i(l-1),:) ;area(i(l-2),:);area(i(l-3),:) ];

== matlab function navigations/monotonic/detectLandMarks/MATLAB Function2 ==
  data: R input; whiteIntensity output; G input; B input
function whiteIntensity  = fcn(R,G,B)
%#codegen
mean(mean((R+G+B)/3,1),2)
whiteIntensity = (R+G+B)- mean(mean((R+G+B)/3,1),2);

== matlab function navigations/monotonic/getPosition/MATLAB Function1 ==
  data: distance input; X output; heading input; rotation input
function X  = fcn(distance,heading,rotation)
X_local = -distance*[sin(rotation(1)); -sin(rotation(2))];
R = [cos(-heading) sin(-heading); -sin(-heading) cos(-heading)];
% X = [R*X_local+offset';distance;heading];
y=R*X_local;
X=[R*X_local'];

== matlab function navigations/monotonic/getPosition/attitudeFix/MATLAB Function ==
  data: PR input; c output; angle input
function c = fcn(PR,angle)
alfa=sqrt((PR(1)-angle(1))^2 +(PR(2)-angle(2))^2);
c=1/cos(alfa);

== matlab function navigations/ImageProcessing 5Color/parseBlues/ParseLandmark/MATLAB Function ==
  data: inputCentroids input; centroids data_store_memory; itt input
function fcn(inputCentroids, itt)
global centroids;
centroids(:,:,itt)=inputCentroids;

== matlab function navigations/ImageProcessing 5Color/findBlue/MATLAB Function1 ==
  data: R input; blueIntensity output; G input; B input
function blueIntensity  = fcn(R,G,B)
%#codegen

blueIntensity = B - R*2/3 - G*2/3;

== matlab function navigations/ImageProcessing 5Color/findBlue/MATLAB Function ==
  data: centroid_largest output; area input; centroid input; bbox_largest output; bbox input
function [centroid_largest, bbox_largest] = selectLargest(area, centroid, bbox)
[y, i] = sort(area);
l=length(area);
bbox_largest = [bbox(i(l),:); bbox(i(l-1),:) ;bbox(i(l-2),:);bbox(i(l-3),:) ];
centroid_largest = [centroid(i(l),:); centroid(i(l-1),:) ;centroid(i(l-2),:);centroid(i(l-3),:) ];

== matlab function navigations/ImageProcessing 5Color/parseBlues/ParseLandmark/Detect Colors/MATLAB Function2 ==
  data: R input; RI output size=[320 240]; GI output size=[320  240]; YI output size=[320  240]; PI output size=[320  240]; G input; B input
function [RI, GI,YI,PI] = fcn(R,G,B)
RI = R - G - B;
GI = G - R - B;
YI = R + G - 3*B;
PI = R + B - 3*G;

== matlab function navigations/ImageProcessing 5Color/parseBlues/ParseLandmark/MATLAB Function2 ==
  data: pos input; itt input; positionData data_store_memory
function writePos(pos, itt)
global positionData;
positionData(itt,:)=pos;

== matlab function navigations/ImageProcessing 5Color/parseBlues/If Action Subsystem1/MATLAB Function1 ==
  data: itt input; positionData data_store_memory
function fcn( itt)
global positionData;
positionData(itt,:)=[-1000 -1000];

== matlab function navigations/ImageProcessing 5Color/parseBlues/ParseLandmark/MATLAB Function1 ==
  data: distance input; X output; heading input; rotation input; offset input; R output; y output
function [X, R,y] = fcn(distance,heading,rotation,offset)
X_local = -distance*[sin(rotation(1)); -sin(rotation(2))];
R = [cos(-heading) sin(-heading); -sin(-heading) cos(-heading)];
% X = [R*X_local+offset';distance;heading];
y=R*X_local;
X=[R*X_local+offset'];

== matlab function navigations/ImageProcessing 5Color/parseBlues/ParseLandmark/attitudeFix/MATLAB Function ==
  data: pitch input; c output; roll input; angle input
function c = fcn(pitch,roll,angle)
alfa=sqrt((pitch-angle(1))^2 +(roll-angle(2))^2);
c=1/cos(alfa);
